simulink model "ysw11_19"  (R2014a)
settings: Solver=ode45  StartTime=0.0  StopTime=10.0  RelTol=1e-3
libraries: commdigbbndpm3 x1
settings Model: Creator=ii  LastModifiedBy=ii
settings SolverCC: ZeroCrossAlgorithm=Adaptive
settings DebuggingCC: UnderspecifiedInitializationDetection=Classic

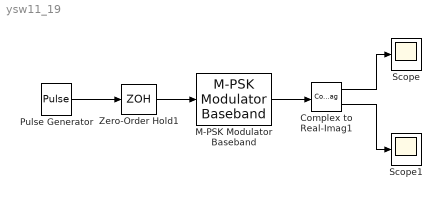
== system ysw11_19 ==
  Complex to Real-Imag1 : ComplexToRealImag
  M-PSK Modulator Baseband : commdigbbndpm3/M-PSK Modulator Baseband  M=32  InType=Integer  Enc=Binary  Mapping=[0:7]  Ph=pi/8  outDtype=double  outWordLen=16  outUDDataType=sfix(16)  outFracLenMode=Best precision  outFracLen=15
  Pulse Generator : DiscretePulseGenerator  PulseType=Time based  Amplitude=3  Period=10  PulseWidth=5
  Scope : Scope
  Scope1 : Scope
  Zero-Order Hold1 : ZeroOrderHold
  wires:
  Complex to Real-Imag1/1 -> Scope/1
  Complex to Real-Imag1/2 -> Scope1/1
  M-PSK Modulator Baseband/1 -> Complex to Real-Imag1/1
  Pulse Generator/1 -> Zero-Order Hold1/1
  Zero-Order Hold1/1 -> M-PSK Modulator Baseband/1
